simulink model "sedemo_resource_allocation"  (Simulink 7.5)
settings: Solver=VariableStepDiscrete  StartTime=0.0  StopTime=10  MaxStep=inf  RelTol=1e-3
undefined symbols (not defined in the file or in its folder): des_figposition
libraries: simeventssink1 x10, simeventsentitymanage1 x4, simeventsgenerators1 x4, simeventsqueue1 x4, simeventsrouting1 x3, simeventsserver1 x2, simulink x2, simeventsinfo x1, simeventsattributes2 x1
CloseFcn:
  | clear  AvgWaitTimeReqsType1;
  | clear  AvgWaitTimeReqsType2;
  | clear  AvgResourcesAvailType1;
  | clear  AvgResourcesAvailType2;
settings Model: Creator=The MathWorks Inc.  ExtModeAutoUpdateStatusClock=off
settings DataIOCC: SaveOutput=off  SaveTime=off
settings OptimizationCC: InitFltsAndDblsToZero=on  EfficientMapNaN2IntZero=off
settings DebuggingCC: AlgebraicLoopMsg=error  SaveWithParameterizedLinksMsg=none  SignalResolutionControl=TryResolveAllWithWarning  SolverPrmCheckMsg=none  StrictBusMsg=Warning
settings GRTTargetCC: TargetFcnLib=ansi_tfl_tmw.mat
settings SimEventsCC: propDiagAttribOutput=1  propDiagFcnCallOutput=1  propDiagStatOutput=0

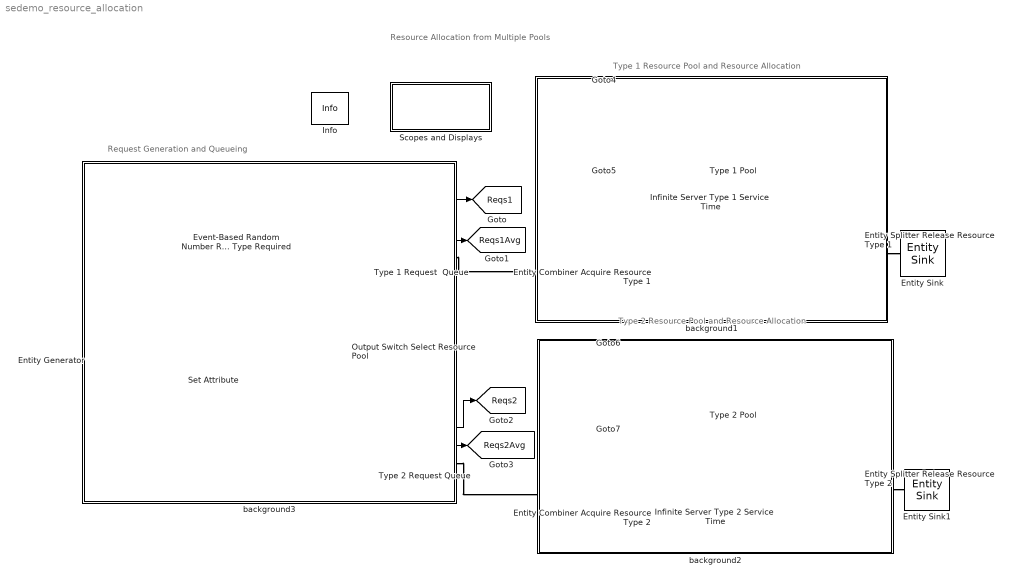
== system sedemo_resource_allocation ==
  note: Resource Allocation from Multiple Pools
  note: Type 1 Resource Pool and Resource Allocation
  note: Type 2 Resource Pool and Resource Allocation
  note: Request Generation and Queueing
  Entity Combiner Acquire Resource Type 1 : simeventsentitymanage1/Entity Combiner  Priority=1  SystemSampleTime=-1  NumberInputPorts=2  RetainComponentEntities=on  AttributeAccessibility=on  TimerAccessibility=on  AttributeCopied=on  TimerCopied=on  StatNumberDeparted=Off  EvaluatedNumPorts=2
  Entity Combiner Acquire Resource Type 2 : simeventsentitymanage1/Entity Combiner  Priority=1  SystemSampleTime=-1  NumberInputPorts=2  RetainComponentEntities=on  AttributeAccessibility=on  TimerAccessibility=on  AttributeCopied=on  TimerCopied=on  StatNumberDeparted=Off  EvaluatedNumPorts=2
  Entity Generator : simeventsgenerators1/Entity Generators/Time-Based Entity Generator  Priority=1  DialogController=des_ddg_create  DialogControllerArgs=DataTag3  SystemSampleTime=-1  GenerateEntitiesUpon=Intergeneration time from dialog  Distribution=Uniform  Minimum=0.001  Maximum=.02  Mean=1  InitialSeed=6765331  Period=.01  PriorityEntityGeneration=300  GenerateEntityAtSimulationStart=on  ResponseWhenBlocked=Pause generation  ResponseWhenUnblocked=Immediate restart  EntityType=Standard  StatNumberDeparted=Off  StatPendingEntity=Off  StatAverageIntergenerationTime=Off
  Entity Sink : simeventssink1/Entity Sink  Priority=1  SystemSampleTime=-1  AvailableForArrivals=on  StatNumberArrived=Off
  Entity Sink1 : simeventssink1/Entity Sink  Priority=1  SystemSampleTime=-1  AvailableForArrivals=on  StatNumberArrived=Off
  Entity Splitter Release Resource Type 1 : simeventsentitymanage1/Entity Splitter  Priority=1  SystemSampleTime=-1  NumberOutputPorts=2  SplitEntityWhen=All entity output ports are not blocked  OutputPortPrecedence=OUT1 port  InitialSeed=56789  ActionUponPortMismatch=Continue  ActionUponBlocking=Discard entity  StatNumberArrived=Off  StatNumberDeparted=Off  EvaluatedNumPorts=2
  Entity Splitter Release Resource Type 2 : simeventsentitymanage1/Entity Splitter  Priority=1  SystemSampleTime=-1  NumberOutputPorts=2  SplitEntityWhen=All entity output ports are not blocked  OutputPortPrecedence=OUT1 port  InitialSeed=56789  ActionUponPortMismatch=Continue  ActionUponBlocking=Discard entity  StatNumberArrived=Off  StatNumberDeparted=Off  EvaluatedNumPorts=2
  Event-Based Random Number Resource Type Required : simeventsgenerators1/Signal Generators/Event-Based Random Number  SystemSampleTime=-1  distribution=Arbitrary discrete  meanExp=1  minUnif=1  maxUnif=1  pOneBern=0.25  pSuccessBino=0.5  numTrialBino=1  meanNorm=0  stdNorm=1  minTri=1  maxTri=3  modeTri=2  thresholdLogn=0  scaleLogn=1  shapeLogn=1  pSuccessGeo=0.5  meanPoiss=1  thresholdLogl=0  scaleLogl=1  thresholdGam=0  scaleGam=1  shapeGam=1  minBeta=0  maxBeta=1  shape1Beta=1  shape2Beta=1  minUnid=0  maxUnid=1  numValueUnid=2  thresholdWbl=0  scaleWbl=1  shapeWbl=1  valueVecCont=[0 1]  cdfVecCont=[0 1]  valueVecDisc=[1 2]  probVecDisc=[0.4 0.6]  seed=345345  IsProcessed=on  isConnected=1
      settings: AttributesFormatString=Prob(Type1,Type2) = %<probVecDisc>
  Infinite Server Type 1 Service  Time : simeventsserver1/Infinite Server  Priority=1  SystemSampleTime=-1  ServiceTimeFrom=Dialog  ServiceTime=.05  AttributeName=ServiceTime  PriorityServiceCompletion=500  EnableTOPort=off  StatNumberDeparted=Off  StatNumberInBlock=Off  StatPendingEntity=Off  StatNumberPending=Off  StatAverageWait=Off  StatNumberTimedout=Off
  Infinite Server Type 2 Service  Time : simeventsserver1/Infinite Server  Priority=1  SystemSampleTime=-1  ServiceTimeFrom=Dialog  ServiceTime=.07  AttributeName=ServiceTime  PriorityServiceCompletion=500  EnableTOPort=off  StatNumberDeparted=Off  StatNumberInBlock=Off  StatPendingEntity=Off  StatNumberPending=Off  StatAverageWait=Off  StatNumberTimedout=Off
  Info : simeventsinfo/Info  SystemSampleTime=-1
  Output Switch Select Resource  Pool : simeventsrouting1/Output Switch  Priority=1  SystemSampleTime=-1  NumberOutputPorts=2  SwitchingCriterion=From attribute  InitialSeed=34567  AttributeName=RequestType  InitialConditionsOpt=off  InitialConditions=1  EntityBufferOpt=off  SpecifyEventPriority=off  PriorityOutputSwitchSelectPort=4100  TimeoutPortOpt=off  StatNumberDeparted=Off  StatNumberTimedOut=Off  StatPendingEntity=Off  StatLastDeparturePort=Off  EvaluatedNumPorts=2
  Scopes and Displays : Subsystem
      mask Display: disp('Scopes and Displays');
  Set Attribute : simeventsattributes2/Set Attribute  Priority=1  DialogController=des_ddg_create  DialogControllerArgs=DataTag16  SystemSampleTime=-1  AttributeFrom=Signal port  AttributeName=RequestType  AttributeTreatAsVector=1  AttributeValue=1  AttributeCreate=on  StatNumberDeparted=Off  EvaluatedAttributeValue={[]}
  Type 1 Pool : Subsystem  mask(Resource Pool Type 1){InitResourcesType1=4}
      mask prompts: InitResourcesType1 "Size of resource pool:"
      mask help: Creates Type 1 resources at the beginning of simulation and stores them for use during the simulation. You can specify the size of this pool by entering a positive finite number for the parameter 'Size of resource pool'.
      settings: AttributesFormatString=Initial Resources = %<InitResourcesType1>
  Type 1 Request  Queue : simeventsqueue1/FIFO Queue  Priority=1  SystemSampleTime=-1  Capacity=inf  EnableTOPort=off  StatNumberDeparted=Off  StatNumberInBlock=On  StatPendingEntity=Off  StatAverageWait=On  StatAverageQueueLength=Off  StatNumberTimedout=Off
  Type 2 Pool : Subsystem  mask(Resource Pool for Type 2){InitResourcesType2=8}
      mask prompts: InitResourcesType2 "Size of resource pool:"
      mask help: Creates type 2 resources at the beginning of simulation and stores them for use during the simulation. You can specify the size of this pool by entering a positive finite number for the parameter 'Size of resource pool'.
      settings: AttributesFormatString=Initial Resources = %<InitResourcesType2>
  Type 2 Request Queue : simeventsqueue1/FIFO Queue  Priority=1  SystemSampleTime=-1  Capacity=inf  EnableTOPort=off  StatNumberDeparted=Off  StatNumberInBlock=On  StatPendingEntity=Off  StatAverageWait=On  StatAverageQueueLength=Off  StatNumberTimedout=Off
  background1 : Subsystem
      mask Display: disp('')
  background2 : Subsystem
      mask Display: disp('')
  background3 : Subsystem
      mask Display: disp('')
  tag scope: AvgRes1=global, AvgRes2=global, Reqs1=global, Reqs1Avg=global, Reqs2=global, Reqs2Avg=global, Res1=global, Res2=global
  wires:
  Type 2 Request Queue/1 -> [Reqs2]
  Event-Based Random Number Resource Type Required/1 -> Set Attribute/1
  Type 1 Request  Queue/1 -> [Reqs1]
  Type 1 Request  Queue/2 -> [Reqs1Avg]
  Type 2 Request Queue/2 -> [Reqs2Avg]
  Type 1 Pool/1(Length) -> [Res1]
  Type 1 Pool/2(Avg Length) -> [AvgRes1]
  Type 2 Pool/1(Length) -> [Res2]
  Type 2 Pool/2(Avg Length) -> [AvgRes2]
  connections:
  Type 1 Pool/RConn1 -- Entity Combiner Acquire Resource Type 1/LConn1
  Type 1 Pool/LConn1 -- Entity Splitter Release Resource Type 1/RConn1
  Entity Combiner Acquire Resource Type 1/RConn1 -- Infinite Server Type 1 Service  Time/LConn1
  Infinite Server Type 1 Service  Time/RConn1 -- Entity Splitter Release Resource Type 1/LConn1
  Entity Splitter Release Resource Type 1/RConn2 -- Entity Sink/LConn1
  Output Switch Select Resource  Pool/RConn1 -- Type 1 Request  Queue/LConn1
  Output Switch Select Resource  Pool/RConn2 -- Type 2 Request Queue/LConn1
  Entity Combiner Acquire Resource Type 2/RConn1 -- Infinite Server Type 2 Service  Time/LConn1
  Entity Splitter Release Resource Type 2/RConn2 -- Entity Sink1/LConn1
  Type 2 Request Queue/RConn1 -- Entity Combiner Acquire Resource Type 2/LConn2
  Infinite Server Type 2 Service  Time/RConn1 -- Entity Splitter Release Resource Type 2/LConn1
  Type 2 Pool/LConn1 -- Entity Splitter Release Resource Type 2/RConn1
  Type 2 Pool/RConn1 -- Entity Combiner Acquire Resource Type 2/LConn1
  Type 1 Request  Queue/RConn1 -- Entity Combiner Acquire Resource Type 1/LConn2
  Set Attribute/RConn1 -- Output Switch Select Resource  Pool/LConn1
  Entity Generator/RConn1 -- Set Attribute/LConn1

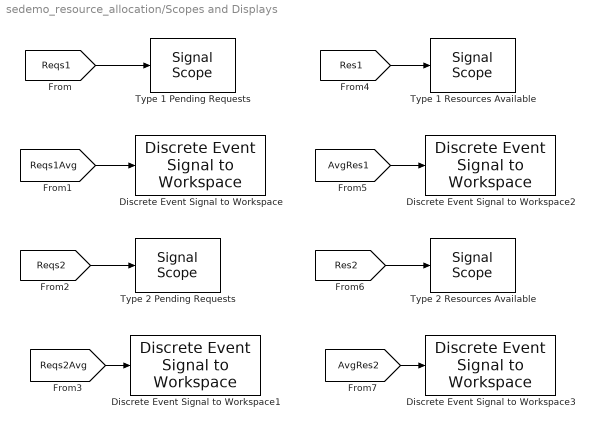
== system sedemo_resource_allocation/Scopes and Displays ==
  Discrete Event Signal to Workspace : simeventssink1/Discrete Event Signal to Workspace  SystemSampleTime=-1  VariableName=AvgWaitTimeReqsType1  SaveFormat=Structure With Time  IsMonitorOnly=off
  Discrete Event Signal to Workspace1 : simeventssink1/Discrete Event Signal to Workspace  SystemSampleTime=-1  VariableName=AvgWaitTimeReqsType2  SaveFormat=Structure With Time  IsMonitorOnly=off
  Discrete Event Signal to Workspace2 : simeventssink1/Discrete Event Signal to Workspace  SystemSampleTime=-1  VariableName=AvgResourcesAvailType1  SaveFormat=Structure With Time  IsMonitorOnly=off
  Discrete Event Signal to Workspace3 : simeventssink1/Discrete Event Signal to Workspace  SystemSampleTime=-1  VariableName=AvgResourcesAvailType2  SaveFormat=Structure With Time  IsMonitorOnly=off
  Type 1 Pending Requests : simeventssink1/Signal Scope  Priority=1  SystemSampleTime=-1  PlotType=Stem  InputType=Signal  NumInputs=1  AttributeNameY=Count  XInputOptionSignal=Event time  XInputOptionEntity=Event time  AttributeNameX=Count  EnableEntityOutport=on  XMin=0  XMax=10  XLimitExceededOption=Keep axis limits unchanged  YLimitExceededOption=Keep axis limits unchanged  AxisGrid=on  AxisLegend=off  LineDisables=""  LineColors="1  0  0"  LineStyles=-  LineMarkers=.  OpenScopeAtSimStart=on  Title=Pending Type 1 Requests  YLabel=Requests  XLabel=Time  FigurePosition=des_figposition([15,5,22,22])  AxisZoom=off  DataStoreOption=Limited  DataPointsLimit=10000  StatNumberArrived=Off  ShowCountPlotted=off  ShowToolbar=on
      settings: YMin=0  YMax=5
  Type 1 Resources Available : simeventssink1/Signal Scope  Priority=1  SystemSampleTime=-1  PlotType=Stair  InputType=Signal  NumInputs=1  AttributeNameY=Count  XInputOptionSignal=Event time  XInputOptionEntity=Event time  AttributeNameX=Count  EnableEntityOutport=on  XMin=0  XMax=10  XLimitExceededOption=Keep axis limits unchanged  YLimitExceededOption=Keep axis limits unchanged  AxisGrid=on  AxisLegend=off  LineDisables=""  LineColors="1  0  0"  LineStyles=-  LineMarkers=.  OpenScopeAtSimStart=on  Title=Type 1 Resources Available  YLabel=Requests  XLabel=Time  FigurePosition=des_figposition([38,5,22,22])  AxisZoom=off  DataStoreOption=Limited  DataPointsLimit=10000  StatNumberArrived=Off  ShowCountPlotted=off  ShowToolbar=on
      settings: YMin=0  YMax=10
  Type 2 Pending Requests : simeventssink1/Signal Scope  Priority=1  SystemSampleTime=-1  PlotType=Stem  InputType=Signal  NumInputs=1  AttributeNameY=Count  XInputOptionSignal=Event time  XInputOptionEntity=Event time  AttributeNameX=Count  EnableEntityOutport=on  XMin=0  XMax=10  XLimitExceededOption=Keep axis limits unchanged  YLimitExceededOption=Keep axis limits unchanged  AxisGrid=on  AxisLegend=off  LineDisables=""  LineColors=b  LineStyles=-  LineMarkers=.  OpenScopeAtSimStart=on  Title=Pending Type 2 Requests  YLabel=Requests  XLabel=Time  FigurePosition=des_figposition([15,28,22,22])  AxisZoom=off  DataStoreOption=Limited  DataPointsLimit=10000  StatNumberArrived=Off  ShowCountPlotted=off  ShowToolbar=on
      settings: YMin=0  YMax=5
  Type 2 Resources Available : simeventssink1/Signal Scope  Priority=1  SystemSampleTime=-1  PlotType=Stair  InputType=Signal  NumInputs=1  AttributeNameY=Count  XInputOptionSignal=Event time  XInputOptionEntity=Event time  AttributeNameX=Count  EnableEntityOutport=on  XMin=0  XMax=10  XLimitExceededOption=Keep axis limits unchanged  YLimitExceededOption=Keep axis limits unchanged  AxisGrid=on  AxisLegend=off  LineDisables=""  LineColors=b  LineStyles=-  LineMarkers=.  OpenScopeAtSimStart=on  Title=Type 2 Resources Available  YLabel=Requests  XLabel=Time  FigurePosition=des_figposition([38,28,22,22])  AxisZoom=off  DataStoreOption=Limited  DataPointsLimit=10000  StatNumberArrived=Off  ShowCountPlotted=off  ShowToolbar=on
      settings: YMin=0  YMax=10
  wires:
  [Reqs1] -> Type 1 Pending Requests/1
  [Reqs1Avg] -> Discrete Event Signal to Workspace/1
  [Reqs2] -> Type 2 Pending Requests/1
  [Reqs2Avg] -> Discrete Event Signal to Workspace1/1
  [Res1] -> Type 1 Resources Available/1
  [AvgRes1] -> Discrete Event Signal to Workspace2/1
  [Res2] -> Type 2 Resources Available/1
  [AvgRes2] -> Discrete Event Signal to Workspace3/1

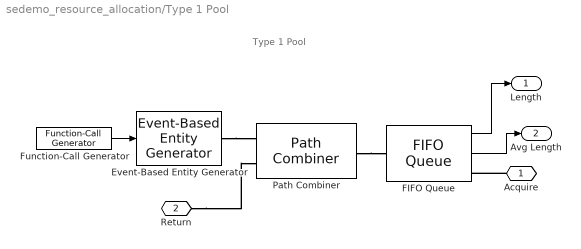
== system sedemo_resource_allocation/Type 1 Pool ==
  note: Type 1 Pool
  Event-Based Entity Generator : simeventsgenerators1/Entity Generators/Event-Based Entity Generator  Priority=1  DialogController=des_ddg_create  DialogControllerArgs=DataTag18  SystemSampleTime=-1  GenerateEntitiesUpon=Function call from port fcn  SignalEdgeType=Rising  SpecifyEventPriority=off  PriorityEntityGeneration=300  GenerateEntityAtSimulationStart=on  AllowBlocking=on  ResponseDuringBlockage=Discard generated entities  EntityType=Blank  StatNumberDeparted=Off  StatPendingEntity=Off  StatAverageIntergenerationTime=Off
  FIFO Queue : simeventsqueue1/FIFO Queue  Priority=1  SystemSampleTime=-1  Capacity=25  EnableTOPort=off  StatNumberDeparted=Off  StatNumberInBlock=On  StatPendingEntity=Off  StatAverageWait=Off  StatAverageQueueLength=On  StatNumberTimedout=Off
  Function-Call Generator : simulink/Ports & Subsystems/Function-Call Generator  sample_time=1e100  numberOfIterations=InitResourcesType1
  Path Combiner : simeventsrouting1/Path Combiner  Priority=1  SystemSampleTime=-1  NumberInputPorts=2  InputPortPrecedence=IN1 port  InitialSeed=45675  SpecifyEventPriority=off  PriorityPathCombinerPortPrecedenceSelection=4100  StatNumberDeparted=Off  StatLastArrivalPort=Off  EvaluatedNumPorts=2
  Acquire : PMIOPort  Port=1  Side=Right
  Return : PMIOPort  Port=2  Side=Left
  Length : Outport  OutDataType=sfix(16)  OutScaling=2^0
  Avg Length : Outport  Port=2  OutDataType=sfix(16)  OutScaling=2^0
  wires:
  Function-Call Generator/1 -> Event-Based Entity Generator/1
  FIFO Queue/1 -> Length/1
  FIFO Queue/2 -> Avg Length/1
  connections:
  Event-Based Entity Generator/RConn1 -- Path Combiner/LConn1
  Path Combiner/RConn1 -- FIFO Queue/LConn1
  Acquire/RConn1 -- FIFO Queue/RConn1
  Return/RConn1 -- Path Combiner/LConn2

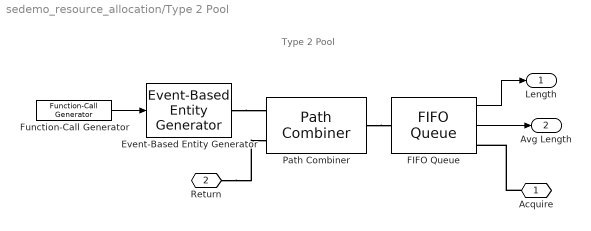
== system sedemo_resource_allocation/Type 2 Pool ==
  note: Type 2 Pool
  Event-Based Entity Generator : simeventsgenerators1/Entity Generators/Event-Based Entity Generator  Priority=1  DialogController=des_ddg_create  DialogControllerArgs=DataTag23  SystemSampleTime=-1  GenerateEntitiesUpon=Function call from port fcn  SignalEdgeType=Rising  SpecifyEventPriority=off  PriorityEntityGeneration=300  GenerateEntityAtSimulationStart=on  AllowBlocking=on  ResponseDuringBlockage=Discard generated entities  EntityType=Blank  StatNumberDeparted=Off  StatPendingEntity=Off  StatAverageIntergenerationTime=Off
  FIFO Queue : simeventsqueue1/FIFO Queue  Priority=1  SystemSampleTime=-1  Capacity=25  EnableTOPort=off  StatNumberDeparted=Off  StatNumberInBlock=On  StatPendingEntity=Off  StatAverageWait=Off  StatAverageQueueLength=On  StatNumberTimedout=Off
  Function-Call Generator : simulink/Ports & Subsystems/Function-Call Generator  sample_time=1e100  numberOfIterations=InitResourcesType2
  Path Combiner : simeventsrouting1/Path Combiner  Priority=1  SystemSampleTime=-1  NumberInputPorts=2  InputPortPrecedence=IN1 port  InitialSeed=45675  SpecifyEventPriority=off  PriorityPathCombinerPortPrecedenceSelection=4100  StatNumberDeparted=Off  StatLastArrivalPort=Off  EvaluatedNumPorts=2
  Acquire : PMIOPort  Port=1  Side=Right
  Return : PMIOPort  Port=2  Side=Left
  Length : Outport  OutDataType=sfix(16)  OutScaling=2^0
  Avg Length : Outport  Port=2  OutDataType=sfix(16)  OutScaling=2^0
  wires:
  Function-Call Generator/1 -> Event-Based Entity Generator/1
  FIFO Queue/2 -> Avg Length/1
  FIFO Queue/1 -> Length/1
  connections:
  Event-Based Entity Generator/RConn1 -- Path Combiner/LConn1
  Path Combiner/RConn1 -- FIFO Queue/LConn1
  Acquire/RConn1 -- FIFO Queue/RConn1
  Return/RConn1 -- Path Combiner/LConn2

== system sedemo_resource_allocation/background1 ==

== system sedemo_resource_allocation/background2 ==

== system sedemo_resource_allocation/background3 ==
